simulink model "satellite3"  (R2025b)
settings: Solver=FixedStepAuto  StartTime=0.0  StopTime=100  FixedStep=dt  MinStep=0.0001  RelTol=1e-3
values from neighbouring files (symbols this model uses):
  A_mw = [ ... (first row only)    [init_params.m]
  A_w = [ ... (first row only)    [init_params.m]
  alpha1 = 0.1    [init_params.m]
  alpha2 = 0.1    [init_params.m]
  angle0 = eAR'    [init_params.m]
  area_d = 4    [init_params.m]
  area_m2 = 0.0127    [init_params.m]
  area_s = 2    [init_params.m]
  ARW_deg_per_sqrt_h = 0.01    [init_params.m]
  B_mw = [ ... (first row only)    [init_params.m]
  bat_bias_on = 0    [init_params.m]
  bat_bias_time = 0    [init_params.m]
  bat_bias_value = 0    [init_params.m]
  bat_cap_on = 0    [init_params.m]
  bat_cap_time = 0    [init_params.m]
  bat_cap_value = 1    [init_params.m]
  beta = 0.3    [init_params.m]
  beta1 = 0.01    [init_params.m]
  beta2 = 0.01    [init_params.m]
  bias0_deg_h = 0.01    [init_params.m]
  C_mw = [ ... (first row only)    [init_params.m]
  Cd = 2.2    [init_params.m]
  Cm = 0.01    [init_params.m]
  cmd_comm = 1    [init_params.m]
  comm_allow = 1    [init_params.m]
  cos_g_max = cos(gamma_max)    [init_params.m]
  Cr = 1.2    [init_params.m]
  cT_deg_on = 0    [init_params.m]
  cT_deg_time = 0    [init_params.m]
  cT_deg_value = 1    [init_params.m]
  cT_delay_on = 0    [init_params.m]
  cT_delay_time = 0    [init_params.m]
  cT_delay_value = 0    [init_params.m]
  cT_drop_on = 0    [init_params.m]
  cT_drop_time = 0    [init_params.m]
  cT_drop_value = 0    [init_params.m]
  cT_lock_on = 0    [init_params.m]
  cT_lock_time = 0    [init_params.m]
  d_c = 2e-5    (= 2e-05)    [init_params.m]
  d_f = 2e-5    (= 2e-05)    [init_params.m]
  D_max = 1    [init_params.m]
  D_thr = 0.4    [init_params.m]
  Delta_D = 0.001    [init_params.m]
  dP_th = 0.05    [init_params.m]
  dss_bias_on = 0    [init_params.m]
  dss_bias_time = 0    [init_params.m]
  dss_bias_value = [0;0;0]    [init_params.m]
  dss_delay_on = 0    [init_params.m]
  dss_delay_time = 0    [init_params.m]
  dss_delay_value = 0    [init_params.m]
  dss_drift_max = 0.1    [init_params.m]
  dss_drift_value = [0;0;0]    [init_params.m]
  dss_drop_on = 0    [init_params.m]
  dss_drop_time = 0    [init_params.m]
  dss_drop_value = [1;0;0]    [init_params.m]
  dss_lock_on = 0    [init_params.m]
  dss_lock_time = 0    [init_params.m]
  dt = 0.1    [init_params.m]
  earth_theta0 = 0    [init_params.m]
  epsilon = 0.01    [init_params.m]
  eT_deg_on = 0    [init_params.m]
  eT_deg_time = 0    [init_params.m]
  eT_deg_value = 1    [init_params.m]
  eT_delay_on = 0    [init_params.m]
  eT_delay_time = 0    [init_params.m]
  eT_delay_value = 0    [init_params.m]
  eT_drop_on = 0    [init_params.m]
  eT_drop_time = 0    [init_params.m]
  eT_drop_value = [0;0;0]    [init_params.m]
  eT_lock_on = 0    [init_params.m]
  eT_lock_time = 0    [init_params.m]
  eta = 0.7    [init_params.m]
  eta_buck = 0.9    [init_params.m]
  eta_et = 0.9    [init_params.m]
  eta_sspa = 0.35    [init_params.m]
  eta_twta = 0.35    [init_params.m]
  f = 2.2e9    (= 2200000000)    [init_params.m]
  f_n_hz = 400    [init_params.m]
  fov = 60*pi/180    (= 1.0471975512)    [init_params.m]
  g0 = 9.80665    [init_params.m]
  G0 = 1366.1    [init_params.m]
  G_sspa_dB = 20    [init_params.m]
  G_twta_dB = 20    [init_params.m]
  Gr_dB = 20    [init_params.m]
  Gt_dB = 3    [init_params.m]
  gyro_bias_on = 0    [init_params.m]
  gyro_bias_time = 0    [init_params.m]
  gyro_bias_value = [0;0;0]    [init_params.m]
  gyro_delay_on = 0    [init_params.m]
  gyro_delay_time = 0    [init_params.m]
  gyro_delay_value = 0    [init_params.m]
  gyro_drift_max = 0.1    [init_params.m]
  gyro_drift_value = [0;0;0]    [init_params.m]
  gyro_drop_on = 0    [init_params.m]
  gyro_drop_time = 0    [init_params.m]
  gyro_drop_value = [0;0;0]    [init_params.m]
  gyro_lock_on = 0    [init_params.m]
  gyro_lock_time = 0    [init_params.m]
  H = 50e3    (= 50000)    [init_params.m]
  h_max = Iw * rpm_max * sqrt(6)    [init_params.m]
  h_ref = 400e3    (= 400000)    [init_params.m]
  I_e = 11    [init_params.m]
  I_gate = 0.5    [init_params.m]
  I_triggle = 8    [init_params.m]
  i_w_max = 2    [init_params.m]
  i_w_min = -2    [init_params.m]
  initial_phase = 0    [init_params.m]
  Isp = 220    [init_params.m]
  Isp_et = 1500    [init_params.m]
  Iw = 0.02    [init_params.m]
  J2 = 1.08262668e-3    (= 0.00108262668)    [init_params.m]
  Jx = 10    [init_params.m]
  Jy = 12    [init_params.m]
  Jz = 8    [init_params.m]
  k_a = 4e-4    (= 0.0004)    [init_params.m]
  k_bias1_deg_h_per_C = 1    [init_params.m]
  k_bias2_deg_h_per_C = 0.0    (= 0)    [init_params.m]
  k_h = -0.05    [init_params.m]
  k_sf1_ppm = 1.0    (= 1)    [init_params.m]
  k_sf2_ppm = 0.0    (= 0)    [init_params.m]
  ... (+207 more)
libraries: matrix_library x25, simulink x14, nesl_utility x4, simulink_extras x3, fl_lib x3, ee_lib x1
(part 5 of 5)

== system satellite3/姿态确定与控制系统/三轴姿态动力学子系统/姿态解算/简化互补滤波器/太敏&地敏/太敏测量/四元数乘法 ==
  Q1 : Inport
  Q2 : Inport  Port=2
  Add : Sum  Inputs=3
  Cross Product : matrix_library/Cross Product
  Demux : Demux
  Demux1 : Demux
  Dot Product : DotProduct  OutDataTypeStr=Inherit: Inherit via internal rule
  Mux : Mux  Inputs=2
  Mux1 : Mux  Inputs=3
  Mux2 : Mux  Inputs=3
  Product : Product
  Product1 : Product
  Product2 : Product
  Sum : Sum  Inputs=|+-
  Q* : Outport
  wires:
  Demux1/4 -> Mux2/3
  Demux1/3 -> Mux2/2
  Demux1/2 -> Mux2/1
  Demux/4 -> Mux1/3
  Demux/3 -> Mux1/2
  Demux/2 -> Mux1/1
  Add/1 -> Mux/2
  Cross Product/1 -> Add/3
  Product1/1 -> Add/1
  Product2/1 -> Add/2
  Dot Product/1 -> Sum/2
  Sum/1 -> Mux/1
  Mux2/1 -> Product1/2, Dot Product/2, Cross Product/2
  Demux1/1 -> Product/2, Product2/1
  Mux1/1 -> Product2/2, Cross Product/1, Dot Product/1
  Demux/1 -> Product/1, Product1/1
  Product/1 -> Sum/1
  Mux/1 -> Q*/1
  Q2/1 -> Demux1/1
  Q1/1 -> Demux/1

== system satellite3/姿态确定与控制系统/三轴姿态动力学子系统/姿态解算/简化互补滤波器/太敏&地敏/太敏预测/hat-s_b ==
  Q1 : Inport
  Q2 : Inport  Port=2
  Add : Sum  Inputs=3
  Cross Product : matrix_library/Cross Product
  Demux : Demux
  Demux1 : Demux
  Mux1 : Mux  Inputs=3
  Mux2 : Mux  Inputs=3
  Product1 : Product
  Product2 : Product
  Q* : Outport
  wires:
  Demux1/4 -> Mux2/3
  Demux1/3 -> Mux2/2
  Demux1/2 -> Mux2/1
  Demux/4 -> Mux1/3
  Demux/3 -> Mux1/2
  Demux/2 -> Mux1/1
  Cross Product/1 -> Add/3
  Product1/1 -> Add/1
  Product2/1 -> Add/2
  Mux2/1 -> Product1/2, Cross Product/2
  Demux1/1 -> Product2/1
  Mux1/1 -> Product2/2, Cross Product/1
  Demux/1 -> Product1/1
  Q2/1 -> Demux1/1
  Q1/1 -> Demux/1
  Add/1 -> Q*/1

== system satellite3/姿态确定与控制系统/三轴姿态动力学子系统/姿态解算/简化互补滤波器/太敏&地敏/太敏预测/共轭 ==
  q : Inport
  -qd1 : Gain  Gain=-1
  -qd2 : Gain  Gain=-1
  -qd3 : Gain  Gain=-1
  Demux : Demux
  Mux : Mux
  q* : Outport
  wires:
  q/1 -> Demux/1
  Mux/1 -> q*/1
  Demux/1 -> Mux/1
  Demux/2 -> -qd1/1
  -qd1/1 -> Mux/2
  Demux/3 -> -qd2/1
  -qd2/1 -> Mux/3
  Demux/4 -> -qd3/1
  -qd3/1 -> Mux/4

== system satellite3/姿态确定与控制系统/三轴姿态动力学子系统/姿态解算/简化互补滤波器/太敏&地敏/太敏预测/向量模长-s_b ==
  u0 : Inport
  u1 : Inport  Port=2
  u2 : Inport  Port=3
  Add : Sum  Inputs=3
  Sqrt : Sqrt
  Square : Math  Operator=square
  Square1 : Math  Operator=square
  Square2 : Math  Operator=square
  |u| : Outport
  wires:
  u0/1 -> Square/1
  u1/1 -> Square1/1
  u2/1 -> Square2/1
  Square/1 -> Add/1
  Square1/1 -> Add/2
  Square2/1 -> Add/3
  Add/1 -> Sqrt/1
  Sqrt/1 -> |u|/1

== system satellite3/姿态确定与控制系统/三轴姿态动力学子系统/姿态解算/简化互补滤波器/太敏&地敏/太敏预测/四元数乘法 ==
  Q1 : Inport
  Q2 : Inport  Port=2
  Add : Sum  Inputs=3
  Cross Product : matrix_library/Cross Product
  Demux : Demux
  Demux1 : Demux
  Dot Product : DotProduct  OutDataTypeStr=Inherit: Inherit via internal rule
  Mux : Mux  Inputs=2
  Mux1 : Mux  Inputs=3
  Mux2 : Mux  Inputs=3
  Product : Product
  Product1 : Product
  Product2 : Product
  Sum : Sum  Inputs=|+-
  Q* : Outport
  wires:
  Q1/1 -> Demux/1
  Q2/1 -> Demux1/1
  Mux/1 -> Q*/1
  Product/1 -> Sum/1
  Demux/1 -> Product1/1, Product/1
  Mux1/1 -> Dot Product/1, Cross Product/1, Product2/2
  Demux1/1 -> Product2/1, Product/2
  Mux2/1 -> Cross Product/2, Dot Product/2, Product1/2
  Sum/1 -> Mux/1
  Dot Product/1 -> Sum/2
  Product2/1 -> Add/2
  Product1/1 -> Add/1
  Cross Product/1 -> Add/3
  Add/1 -> Mux/2
  Demux/2 -> Mux1/1
  Demux/3 -> Mux1/2
  Demux/4 -> Mux1/3
  Demux1/2 -> Mux2/1
  Demux1/3 -> Mux2/2
  Demux1/4 -> Mux2/3

== system satellite3/姿态确定与控制系统/三轴姿态动力学子系统/姿态解算/简化互补滤波器/太敏&地敏/太敏预测/太敏噪声 ==
  note: 先用正弦伪噪声，再考虑换成随机噪声
  1 : simulink/Sources/Band-Limited White Noise  Cov=[0.1]  Ts=0.1  seed=[23341]
  Mux : Mux  Inputs=3
  Sine Wave : Sin  Amplitude=sigma_sun  Frequency=2*pi*1  SampleTime=0
  Sine Wave1 : Sin  Amplitude=sigma_sun  Frequency=2*pi*1  SampleTime=0
  Sine Wave2 : Sin  Amplitude=sigma_sun  Frequency=2*pi*1  SampleTime=0
  noise : Outport
  wires:
  Sine Wave/1 -> Mux/1
  Mux/1 -> noise/1
  Sine Wave1/1 -> Mux/2
  Sine Wave2/1 -> Mux/3

== system satellite3/姿态确定与控制系统/三轴姿态动力学子系统/姿态解算/简化互补滤波器/太敏&地敏/太敏预测/太敏故障 ==
  原值 : Inport
  Add : Sum  Inputs=+++++
  Sum : Sum  Inputs=|++
  偏差故障 : Subsystem
  延迟故障 : Subsystem
  掉线故障 : Subsystem
  漂移故障 : Subsystem
  锁死故障 : Subsystem
  故障值 : Outport
  wires:
  延迟故障/1(故障值注入) -> Add/5
  掉线故障/1(故障值注入) -> Add/4
  锁死故障/1(故障值注入) -> Add/3
  漂移故障/1(故障值注入) -> Add/2
  偏差故障/1(故障值注入) -> Add/1
  Add/1 -> Sum/2
  Sum/1 -> 故障值/1
  原值/1 -> Sum/1, 锁死故障/1(原值), 掉线故障/1(原值), 延迟故障/1(原值)

== system satellite3/姿态确定与控制系统/三轴姿态动力学子系统/姿态解算/简化互补滤波器/太敏&地敏/地敏测量/hat-s_b/向量模长-T ==
  u : Inport
  Add : Sum  Inputs=+++
  Demux : Demux  Outputs=3
  Sqrt : Sqrt
  Square : Math  Operator=square
  Square1 : Math  Operator=square
  Square2 : Math  Operator=square
  |u| : Outport
  wires:
  Demux/2 -> Square1/1
  Demux/3 -> Square2/1
  Square/1 -> Add/1
  Square1/1 -> Add/2
  Square2/1 -> Add/3
  Add/1 -> Sqrt/1
  Sqrt/1 -> |u|/1
  Demux/1 -> Square/1
  u/1 -> Demux/1

== system satellite3/姿态确定与控制系统/三轴姿态动力学子系统/姿态解算/简化互补滤波器/太敏&地敏/地敏预测/hat-s_b/向量模长-T ==
  u : Inport
  Add : Sum  Inputs=+++
  Demux : Demux  Outputs=3
  Sqrt : Sqrt
  Square : Math  Operator=square
  Square1 : Math  Operator=square
  Square2 : Math  Operator=square
  |u| : Outport
  wires:
  Demux/2 -> Square1/1
  Demux/3 -> Square2/1
  Square/1 -> Add/1
  Square1/1 -> Add/2
  Square2/1 -> Add/3
  Add/1 -> Sqrt/1
  Sqrt/1 -> |u|/1
  Demux/1 -> Square/1
  u/1 -> Demux/1

== system satellite3/姿态确定与控制系统/三轴姿态动力学子系统/姿态解算/简化互补滤波器/太敏&地敏/太敏预测/太敏故障/偏差故障 ==
  使能*幅度 : Gain  Gain=dss_bias_on*dss_bias_value
  注入时间 : Step  Time=dss_bias_time  SampleTime=0
  故障值注入 : Outport
  wires:
  使能*幅度/1 -> 故障值注入/1
  注入时间/1 -> 使能*幅度/1

== system satellite3/姿态确定与控制系统/三轴姿态动力学子系统/姿态解算/简化互补滤波器/太敏&地敏/太敏预测/太敏故障/延迟故障 ==
  原值 : Inport
  Delay : Delay  DelayLength=dss_delay_value
  Switch : Switch  Criteria=u2 > Threshold  Threshold=0.5  SaturateOnIntegerOverflow=off  InputSameDT=off
  使能 : Gain  Gain=dss_delay_on
  抵消 : Sum  Inputs=|+-
  注入时间 : Step  Time=dss_delay_time  SampleTime=0
  故障值注入 : Outport
  wires:
  Delay/1 -> Switch/1
  Switch/1 -> 抵消/1
  抵消/1 -> 故障值注入/1
  原值/1 -> 抵消/2, Delay/1, Switch/3
  注入时间/1 -> 使能/1
  使能/1 -> Switch/2

== system satellite3/姿态确定与控制系统/三轴姿态动力学子系统/姿态解算/简化互补滤波器/太敏&地敏/太敏预测/太敏故障/掉线故障 ==
  原值 : Inport
  Switch : Switch  Criteria=u2 > Threshold  Threshold=0.5  SaturateOnIntegerOverflow=off  InputSameDT=off
  Zero : Constant  Value=dss_drop_value  OutDataTypeStr=Inherit: Inherit via back propagation
  使能 : Gain  Gain=dss_drop_on
  抵消 : Sum  Inputs=|+-
  注入时间 : Step  Time=dss_drop_time  SampleTime=0
  故障值注入 : Outport
  wires:
  使能/1 -> Switch/2
  注入时间/1 -> 使能/1
  原值/1 -> Switch/3, 抵消/2
  抵消/1 -> 故障值注入/1
  Switch/1 -> 抵消/1
  Zero/1 -> Switch/1

== system satellite3/姿态确定与控制系统/三轴姿态动力学子系统/姿态解算/简化互补滤波器/太敏&地敏/太敏预测/太敏故障/漂移故障 ==
  使能*幅度 : Gain  Gain=dss_bias_on*dss_drift_value
  注入时间 : simulink/Sources/Ramp  slope=1  start=dss_drift_time  InitialOutput=0
  限幅 : Saturate  UpperLimit=dss_drift_max  LowerLimit=-dss_drift_max
  故障值注入 : Outport
  wires:
  限幅/1 -> 故障值注入/1
  注入时间/1 -> 使能*幅度/1
  使能*幅度/1 -> 限幅/1

== system satellite3/姿态确定与控制系统/三轴姿态动力学子系统/姿态解算/简化互补滤波器/太敏&地敏/太敏预测/太敏故障/锁死故障 ==
  原值 : Inport
  Switch : Switch  Criteria=u2 > Threshold  Threshold=0.5  SaturateOnIntegerOverflow=off  InputSameDT=off
  上一值 : UnitDelay  SampleTime=-1  HasFrameUpgradeWarning=on
  使能 : Gain  Gain=dss_lock_on
  抵消 : Sum  Inputs=|+-
  注入时间 : Step  Time=dss_lock_time  SampleTime=0
  故障值注入 : Outport
  wires:
  Switch/1 -> 抵消/1, 上一值/1
  原值/1 -> 抵消/2, Switch/3
  使能/1 -> Switch/2
  上一值/1 -> Switch/1
  抵消/1 -> 故障值注入/1
  注入时间/1 -> 使能/1

== matlab function satellite3/姿态确定与控制系统/三轴姿态动力学子系统/姿态解算/欧拉角 ==
  data: Q input double size=4; angle output double size=3
function angle = eulerangle(Q)

quat = quaternion(Q(1),Q(2),Q(3),Q(4));
eAR = euler(quat, 'ZYX', 'frame');% eulerAngles,Rad
angle = eAR';   % 初始角度

== matlab function satellite3/环境与动力学子系统/J2000模型/J2000_r_sun ==
  data: r_sun_GCI_km output; t input; utc0_jd input; s_hat output
function [r_sun_GCI_km,s_hat] = sunJ2000_GCI(t, utc0_jd)
%#codegen
% sunVectorJ2000_GCI
%
% 功能：
%   计算地心到太阳的位置向量，坐标系为近似 J2000/GCI 惯性系
%
% 输入：
%   t    : 仿真时间（秒），从起始历元 utc0 开始累计
%   utc0 : 起始时间（datetime 类型，UTC）
%
% 输出：
%   r_sun_GCI_km : 太阳在 GCI(J2000近似)坐标系下的位置向量 [km]
%   s_hat        : 指向太阳的单位向量
%   JD_utc       : 当前时刻 UTC 儒略日
%   T            : 相对于 J2000 的儒略世纪
%
% 说明：
%   本算法采用 Meeus 太阳位置近似公式，工程精度足够用于
%   航天器姿态控制、太阳照射判断等仿真。
%
%   此处 GCI 近似为 J2000 平赤道平春分点坐标系。

%% 常数
AU_km = 149597870.7;    % 天文单位 [km]

%% 计算当前UTC儒略日
JD_utc = utc0_jd + t/86400.0;  % 秒转天

%% 计算 J2000 起算的儒略世纪
T = (JD_utc - 2451545.0) / 36525.0;

%% ================= 太阳轨道参数 =================

% 太阳平黄经（deg）
L0 = 280.46646 + 36000.76983*T + 0.0003032*T*T;

% 太阳平近点角（deg）
M  = 357.52911 + 35999.05029*T - 0.0001537*T*T;

% 角度归一化到 [0,360)
L0 = wrapTo360(L0);
M  = wrapTo360(M);

% 地球轨道偏心率
e = 0.016708634 - 0.000042037*T - 0.0000001267*T*T;

% 转弧度用于三角函数
Mrad = deg2rad(M);

% 太阳中心差（deg）
C = (1.914602 - 0.004817*T - 0.000014*T*T) * sin(Mrad) + ...
    (0.019993 - 0.000101*T) * sin(2*Mrad) + ...
     0.000289 * sin(3*Mrad);

% 太阳真黄经（deg）
lambda = wrapTo360(L0 + C);

% 太阳真近点角（deg）
nu = wrapTo360(M + C);

% 地日距离（单位 AU）
nurad = deg2rad(nu);
R_AU = (1.000001018*(1 - e*e)) / (1 + e*cos(nurad));

%% ================= 黄道系 -> 赤道系 =================

% 黄赤交角（deg）
eps = 23.439291 - 0.0130042*T - 1.64e-7*T*T + 5.04e-7*T*T*T;

% 转弧度
lamrad = deg2rad(lambda);
epsrad = deg2rad(eps);

% 在黄道坐标系下太阳向量
x = R_AU * cos(lamrad);
y = R_AU * sin(lamrad) * cos(epsrad);
z = R_AU * sin(lamrad) * sin(epsrad);

% 转换为 km
r_sun_GCI_km = AU_km * [x; y; z];

%% 计算单位向量
rnorm = sqrt(r_sun_GCI_km(1)^2 + r_sun_GCI_km(2)^2 + r_sun_GCI_km(3)^2);

if rnorm > 0
    s_hat = r_sun_GCI_km / rnorm;
else
    s_hat = [0;0;0];
end

end


%% ================= 辅助函数 =================

function JD = datetimeToJulianDateUTC(dt)
% 将 UTC datetime 转换为儒略日 JD

y = year(dt);
m = month(dt);
d = day(dt);
hh = hour(dt);
mm = minute(dt);
ss = second(dt);

% 计算一天中的小数部分
frac = (hh + (mm + ss/60.0)/60.0) / 24.0;
D = double(d) + frac;

% 若月份为1或2月，需要进行转换
if m <= 2
    y = y - 1;
    m = m + 12;
end

A = floor(y/100);
B = 2 - A + floor(A/4);

JD = floor(365.25*(y + 4716)) + ...
     floor(30.6001*(m + 1)) + ...
     D + B - 1524.5;

end


function ang = wrapTo360(ang)
% 将角度归一化到 [0,360)

ang = mod(ang, 360.0);

if ang < 0
    ang = ang + 360.0;
end

end

== matlab function satellite3/环境与动力学子系统/惯性转轨道 ==
  data: i input; RA input; TA input; w input; r input; r_ss output
function r_ss  =  fcn(i,RA,TA,w,r)
u = w + TA;
a = [0 1 0;0 0 -1;-1 0 0];
A = [cos(u) sin(u) 0;-sin(u) cos(u) 0;0 0 1];
B = [1 0 0;0 cos(i) sin(i);0 -sin(i) cos(i)];
C = [cos(RA) sin(RA) 0;-sin(RA) cos(RA) 0;0 0 1];
r_ss = a*A*B*C*r;
% Toi  =  [-sin(u)*cos(RA)-cos(u)*cos(i)*sin(RA),    -sin(u)*sin(RA) +cos(u)*cos(i)*cos(RA),   cos(u)*sin(i);
%         -sin(i)*sin(RA),                         sin(i)*cos(RA),                          -cos(i);
%         -cos(u)*cos(RA) +sin(u)*cos(i)*sin(RA),   -cos(u)*sin(RA)-sin(u)*cos(i)*cos(RA),    -sin(u)*sin(i)];
%由惯性坐标系到轨道坐标系的转换矩阵

== matlab function satellite3/姿态确定与控制系统/重力梯度力矩/地心转轨道 ==
  data: r input; i input; RA input; TA input; w input; r_o output
function r_o = fcn(r,i,RA,TA,w)
u = w + TA;
a = [0 1 0;
    0 0 -1;
    -1 0 0
];
A=[cos(u) sin(u) 0;-sin(u) cos(u) 0;0 0 1];
B=[1 0 0;0 cos(i) sin(i);0 -sin(i) cos(i)];
C=[cos(RA) sin(RA) 0;-sin(RA) cos(RA) 0;0 0 1];
r_o=a*A*B*C*r;
% Toi = [-sin(u)*cos(RA)-cos(u)*cos(i)*sin(RA),    -sin(u)*sin(RA)+cos(u)*cos(i)*cos(RA),   cos(u)*sin(i);
%         -sin(i)*sin(RA),                         sin(i)*cos(RA),                          -cos(i);
%         -cos(u)*cos(RA)+sin(u)*cos(i)*sin(RA),   -cos(u)*sin(RA)-sin(u)*cos(i)*cos(RA),    -sin(u)*sin(i)];
%由惯性坐标系到轨道坐标系的转换矩阵
